simulink model "simulink_model_1"  (R2022a)
settings: Solver=VariableStepAuto  StartTime=0.0  StopTime=020.0  RelTol=1e-3
values from neighbouring files (symbols this model uses):
  Td = 0.2    [RTII_MatlabUe1.m]    (also in RTII_MatlabUe3.m = 0.1)
undefined symbols (not defined in the file or in its folder): denRt, numRt
libraries: cstblocks x2
settings Model: Creator=valnim  LastModifiedBy=valni
settings SolverCC: AlgebraicLoopSolver=TrustRegion
settings DebuggingCC: UnconnectedInputMsg=warning  UnconnectedOutputMsg=warning  UnconnectedLineMsg=warning  SFMachineParentedDataDiag=warning
settings RTWCC: DLArmComputeVersion=19.05

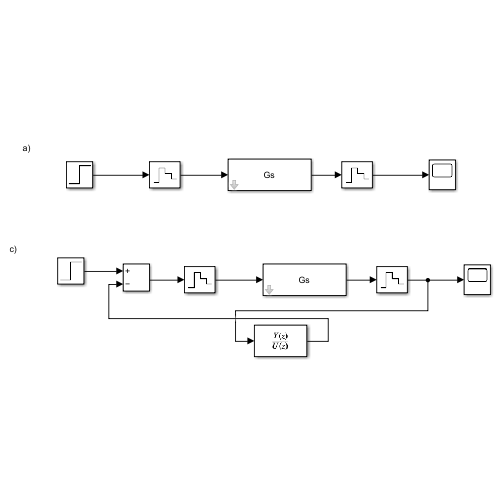
[thumbnail: Simulink's stored preview of the top-level diagram]
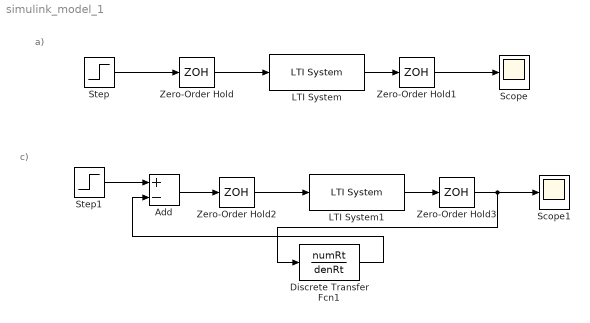
== system simulink_model_1 ==
  note: a)
  note: c)
  Add : Sum  Inputs=+-
  Discrete Transfer Fcn1 : DiscreteTransferFcn  Numerator=numRt  Denominator=denRt  SampleTime=Td
  LTI System : cstblocks/LTI System  sys=Gs  IC=[]
  LTI System1 : cstblocks/LTI System  sys=Gs  IC=[]
  Scope : Scope
  Scope1 : Scope
  Step : Step  Time=0  SampleTime=0
  Step1 : Step  Time=0  SampleTime=0
  Zero-Order Hold{,1..3} (4 alike) : ZeroOrderHold  SampleTime=Td
  wires:
  Step/1 -> Zero-Order Hold/1
  Zero-Order Hold/1 -> LTI System/1
  LTI System/1 -> Zero-Order Hold1/1
  Zero-Order Hold1/1 -> Scope/1
  Zero-Order Hold2/1 -> LTI System1/1
  LTI System1/1 -> Zero-Order Hold3/1
  Step1/1 -> Add/1
  Add/1 -> Zero-Order Hold2/1
  Zero-Order Hold3/1 -> Discrete Transfer Fcn1/1, Scope1/1
  Discrete Transfer Fcn1/1 -> Add/2
